simulink subsystem "Tranfsform_Linear_Gains_To_World"  (R2023a)
settings: Solver=VariableStepAuto  StartTime=0.0  StopTime=10.0  RelTol=1e-3

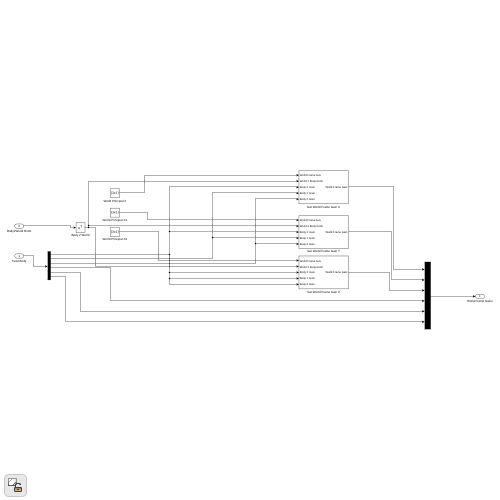
[thumbnail: Simulink's stored preview of the top-level diagram]
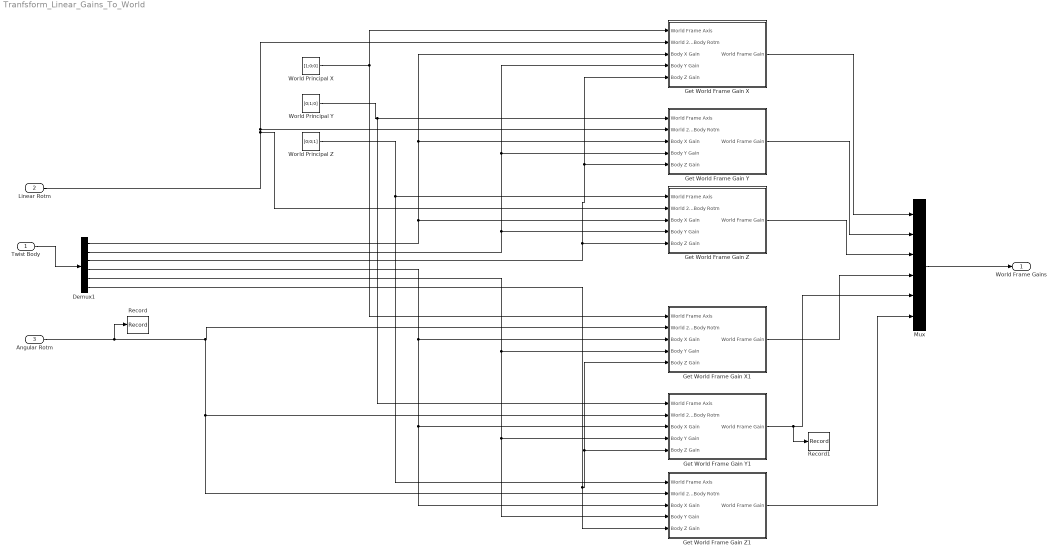
== system Tranfsform_Linear_Gains_To_World ==
  Twist Body : Inport
  Linear Rotm : Inport  Port=2
  Angular Rotm : Inport  Port=3
  Demux1 : Demux  Outputs=6
  Get World Frame Gain X : Subsystem
  Get World Frame Gain X1 : Subsystem
  Get World Frame Gain Y : Subsystem
  Get World Frame Gain Y1 : Subsystem
  Get World Frame Gain Z : Subsystem
  Get World Frame Gain Z1 : Subsystem
  Mux : Mux  Inputs=6
  Record : Record  FileSettingsInternal="{\"entries\":[{\"content\":{\"excelSettings\":{\"content\":{},\"type\":\"Streamout.ExcelSettings\"}},\"type\":\"Streamout.FileSettingStorage\",\"uuid\":\"\"}],\"packageUris\":[\"http:\\/\\/schema.mathworks.com\\/mf0\\/streamout_blocks\\/R2020a\"],\"version\":\"1.0\"}"  Layout=[1 1]  SignalsInternal="{\"entries\":[{\"content\":{\"signals\":[{\"content\":{\"blockPath\":[],\"dimensions\":[3,3],\"domain\":\"\",\"hasChildren\":true,\"lineColor\":\"#7e2f8e\",\"port\":1,\"signalID\":164792,\"signalName\":\"Angular Rotm\"},\"type\":\"RecordBlkView.Signal\",\"uuid\":\"\"},{\"content\":{\"blockPath\":[],\"channel\":[1,1],\"dimensions\":[3,3],\"domain\":\"\",\"lineColor\":\"#77ac30\",\"parentID\":164792,\"plots\":[1],\"port\":1,\"signalID\":164793,\"signalName\":\"An ...(+1923 chars)"  VisualizationBindings="{\"sparklinesplugin\":{\"info\":[{\"bindingParametersList\":[],\"subplotID\":1}]}}"
  Record1 : Record  FileSettingsInternal="{\"entries\":[{\"content\":{\"excelSettings\":{\"content\":{},\"type\":\"Streamout.ExcelSettings\"}},\"type\":\"Streamout.FileSettingStorage\",\"uuid\":\"\"}],\"packageUris\":[\"http:\\/\\/schema.mathworks.com\\/mf0\\/streamout_blocks\\/R2020a\"],\"version\":\"1.0\"}"  Layout=[1 1]  SignalsInternal="{\"entries\":[{\"content\":{\"signals\":[{\"content\":{\"blockPath\":[],\"dimensions\":[1],\"domain\":\"\",\"lineColor\":\"#a2142f\",\"plots\":[1],\"port\":1,\"signalID\":164815,\"signalName\":\"Get World Frame Gain Y1\"},\"type\":\"RecordBlkView.Signal\",\"uuid\":\"\"}]},\"type\":\"RecordBlkView.InputSignals\",\"uuid\":\"\"}],\"packageUris\":[\"http:\\/\\/schema.mathworks.com\\/mf0\\/streamout_blocks\\/R2020a\"],\"version\":\"1.0\"}"  VisualizationBindings="{\"sparklinesplugin\":{\"info\":[{\"bindingParametersList\":[],\"subplotID\":1}]}}"
  World Principal X : Constant  Value=[1;0;0]
  World Principal Y : Constant  Value=[0;1;0]
  World Principal Z : Constant  Value=[0;0;1]
  World Frame Gains : Outport
  wires:
  Twist Body/1 -> Demux1/1
  Demux1/1 -> Get World Frame Gain X/3(Body X Gain), Get World Frame Gain Y/3(Body X Gain), Get World Frame Gain Z/3(Body X Gain)
  Demux1/2 -> Get World Frame Gain X/4(Body Y Gain), Get World Frame Gain Y/4(Body Y Gain), Get World Frame Gain Z/4(Body Y Gain)
  Demux1/3 -> Get World Frame Gain X/5(Body Z Gain), Get World Frame Gain Y/5(Body Z Gain), Get World Frame Gain Z/5(Body Z Gain)
  Linear Rotm/1 -> Get World Frame Gain X/2(World 2 Body Rotm), Get World Frame Gain Y/2(World 2 Body Rotm), Get World Frame Gain Z/2(World 2 Body Rotm)
  Mux/1 -> World Frame Gains/1
  Get World Frame Gain X/1(World Frame Gain) -> Mux/1
  Get World Frame Gain Y/1(World Frame Gain) -> Mux/2
  Get World Frame Gain Z/1(World Frame Gain) -> Mux/3
  Get World Frame Gain Y1/1(World Frame Gain) -> Mux/5, Record1/1
  Demux1/5 -> Get World Frame Gain Y1/4(Body Y Gain), Get World Frame Gain Z1/4(Body Y Gain), Get World Frame Gain X1/4(Body Y Gain)
  Demux1/4 -> Get World Frame Gain Y1/3(Body X Gain), Get World Frame Gain Z1/3(Body X Gain), Get World Frame Gain X1/3(Body X Gain)
  World Principal Z/1 -> Get World Frame Gain Z/1(World Frame Axis), Get World Frame Gain Z1/1(World Frame Axis)
  World Principal X/1 -> Get World Frame Gain X1/1(World Frame Axis), Get World Frame Gain X/1(World Frame Axis)
  Get World Frame Gain Z1/1(World Frame Gain) -> Mux/6
  World Principal Y/1 -> Get World Frame Gain Y1/1(World Frame Axis), Get World Frame Gain Y/1(World Frame Axis)
  Demux1/6 -> Get World Frame Gain Y1/5(Body Z Gain), Get World Frame Gain X1/5(Body Z Gain), Get World Frame Gain Z1/5(Body Z Gain)
  Get World Frame Gain X1/1(World Frame Gain) -> Mux/4
  Angular Rotm/1 -> Get World Frame Gain Y1/2(World 2 Body Rotm), Get World Frame Gain Z1/2(World 2 Body Rotm), Get World Frame Gain X1/2(World 2 Body Rotm), Record/1

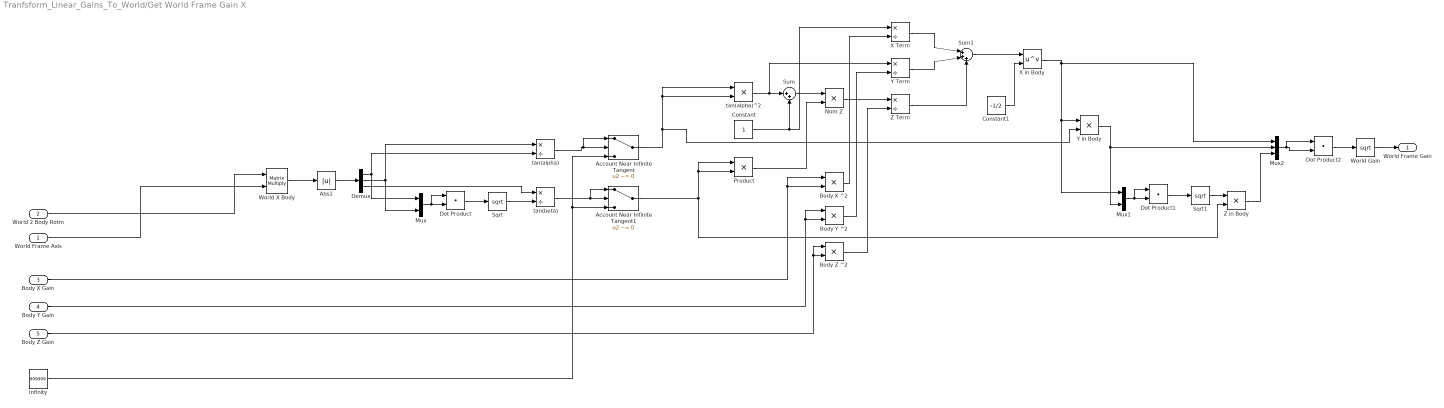
== system Tranfsform_Linear_Gains_To_World/Get World Frame Gain X ==
  World Frame Axis : Inport
  World 2 Body Rotm : Inport  Port=2
  Body X Gain : Inport  Port=3
  Body Y Gain : Inport  Port=4
  Body Z Gain : Inport  Port=5
  Abs1 : Abs  SaturateOnIntegerOverflow=off
  Account Near Infinite Tangent : Switch  Criteria=u2 ~= 0  SaturateOnIntegerOverflow=off  InputSameDT=off
  Account Near Infinite Tangent1 : Switch  Criteria=u2 ~= 0  SaturateOnIntegerOverflow=off  InputSameDT=off
  Body X ^2 : Product
  Body Y ^2 : Product
  Body Z ^2 : Product
  Constant : Constant
  Constant1 : Constant  Value=-1/2
  Demux : Demux  Outputs=3
  Dot Product : DotProduct  OutDataTypeStr=Inherit: Inherit via internal rule
  Dot Product1 : DotProduct  OutDataTypeStr=Inherit: Inherit via internal rule
  Dot Product2 : DotProduct  OutDataTypeStr=Inherit: Inherit via internal rule
  Infinity : Constant  Value=999999
  Mux : Mux  Inputs=2
  Mux1 : Mux  Inputs=2
  Mux2 : Mux  Inputs=3
  Num Z : Product
  Product : Product
  Sqrt : Sqrt
  Sqrt1 : Sqrt
  Sum : Sum  Inputs=|++
  Sum1 : Sum  Inputs=|+++
  World Gain : Sqrt
  World X Body : Product  Multiplication=Matrix(*)
  X Term : Product  Inputs=*/
  X in Body : Math  Operator=pow
  Y Term : Product  Inputs=*/
  Y in Body : Product
  Z Term : Product  Inputs=*/
  Z in Body : Product
  tan(alpha) : Product  Inputs=*/
  tan(alpha)^2 : Product
  tan(beta) : Product  Inputs=*/
  World Frame Gain : Outport
  wires:
  Account Near Infinite Tangent1/1 -> Z in Body/2, Product/1, Product/2
  tan(beta)/1 -> Account Near Infinite Tangent1/2, Account Near Infinite Tangent1/1
  Infinity/1 -> Account Near Infinite Tangent/3, Account Near Infinite Tangent1/3
  tan(alpha)/1 -> Account Near Infinite Tangent/2, Account Near Infinite Tangent/1
  Account Near Infinite Tangent/1 -> Y in Body/2, tan(alpha)^2/2, tan(alpha)^2/1
  World X Body/1 -> Abs1/1
  Sum/1 -> Num Z/1
  Mux2/1 -> Dot Product2/2, Dot Product2/1
  Demux/2 -> tan(alpha)/1, Mux/2
  Dot Product1/1 -> Sqrt1/1
  Constant/1 -> Sum/2, X Term/1
  Z in Body/1 -> Mux2/3
  Body X ^2/1 -> X Term/2
  Body X Gain/1 -> Body X ^2/1, Body X ^2/2
  Product/1 -> Num Z/2
  X Term/1 -> Sum1/1
  Abs1/1 -> Demux/1
  Dot Product/1 -> Sqrt/1
  Y Term/1 -> Sum1/2
  Body Z Gain/1 -> Body Z ^2/1, Body Z ^2/2
  Sqrt/1 -> tan(beta)/2
  Y in Body/1 -> Mux1/2, Mux2/2
  Sqrt1/1 -> Z in Body/1
  Body Y Gain/1 -> Body Y ^2/1, Body Y ^2/2
  Demux/1 -> tan(alpha)/2, Mux/1
  Body Z ^2/1 -> Z Term/2
  Num Z/1 -> Z Term/1
  Body Y ^2/1 -> Y Term/2
  X in Body/1 -> Y in Body/1, Mux1/1, Mux2/1
  Mux/1 -> Dot Product/1, Dot Product/2
  Constant1/1 -> X in Body/2
  Z Term/1 -> Sum1/3
  World Gain/1 -> World Frame Gain/1
  tan(alpha)^2/1 -> Sum/1, Y Term/1
  World 2 Body Rotm/1 -> World X Body/1
  Mux1/1 -> Dot Product1/1, Dot Product1/2
  Sum1/1 -> X in Body/1
  Dot Product2/1 -> World Gain/1
  World Frame Axis/1 -> World X Body/2
  Demux/3 -> tan(beta)/1

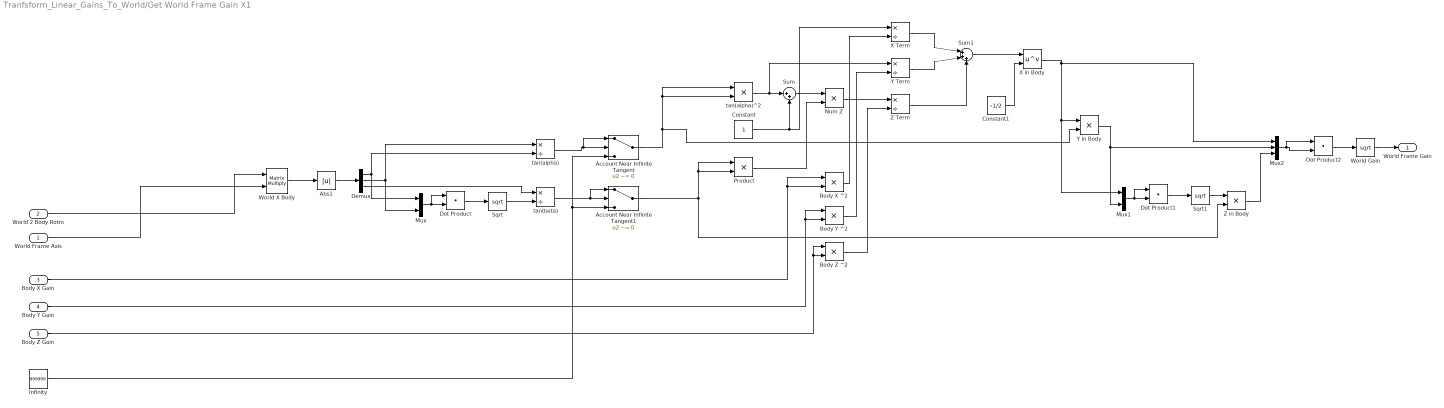
== system Tranfsform_Linear_Gains_To_World/Get World Frame Gain X1 ==
  World Frame Axis : Inport
  World 2 Body Rotm : Inport  Port=2
  Body X Gain : Inport  Port=3
  Body Y Gain : Inport  Port=4
  Body Z Gain : Inport  Port=5
  Abs1 : Abs  SaturateOnIntegerOverflow=off
  Account Near Infinite Tangent : Switch  Criteria=u2 ~= 0  SaturateOnIntegerOverflow=off  InputSameDT=off
  Account Near Infinite Tangent1 : Switch  Criteria=u2 ~= 0  SaturateOnIntegerOverflow=off  InputSameDT=off
  Body X ^2 : Product
  Body Y ^2 : Product
  Body Z ^2 : Product
  Constant : Constant
  Constant1 : Constant  Value=-1/2
  Demux : Demux  Outputs=3
  Dot Product : DotProduct  OutDataTypeStr=Inherit: Inherit via internal rule
  Dot Product1 : DotProduct  OutDataTypeStr=Inherit: Inherit via internal rule
  Dot Product2 : DotProduct  OutDataTypeStr=Inherit: Inherit via internal rule
  Infinity : Constant  Value=999999
  Mux : Mux  Inputs=2
  Mux1 : Mux  Inputs=2
  Mux2 : Mux  Inputs=3
  Num Z : Product
  Product : Product
  Sqrt : Sqrt
  Sqrt1 : Sqrt
  Sum : Sum  Inputs=|++
  Sum1 : Sum  Inputs=|+++
  World Gain : Sqrt
  World X Body : Product  Multiplication=Matrix(*)
  X Term : Product  Inputs=*/
  X in Body : Math  Operator=pow
  Y Term : Product  Inputs=*/
  Y in Body : Product
  Z Term : Product  Inputs=*/
  Z in Body : Product
  tan(alpha) : Product  Inputs=*/
  tan(alpha)^2 : Product
  tan(beta) : Product  Inputs=*/
  World Frame Gain : Outport
  wires:
  Account Near Infinite Tangent1/1 -> Z in Body/2, Product/1, Product/2
  tan(beta)/1 -> Account Near Infinite Tangent1/2, Account Near Infinite Tangent1/1
  Infinity/1 -> Account Near Infinite Tangent/3, Account Near Infinite Tangent1/3
  tan(alpha)/1 -> Account Near Infinite Tangent/2, Account Near Infinite Tangent/1
  Account Near Infinite Tangent/1 -> Y in Body/2, tan(alpha)^2/2, tan(alpha)^2/1
  World X Body/1 -> Abs1/1
  Sum/1 -> Num Z/1
  Mux2/1 -> Dot Product2/2, Dot Product2/1
  Demux/2 -> tan(alpha)/1, Mux/2
  Dot Product1/1 -> Sqrt1/1
  Constant/1 -> Sum/2, X Term/1
  Z in Body/1 -> Mux2/3
  Body X ^2/1 -> X Term/2
  Body X Gain/1 -> Body X ^2/1, Body X ^2/2
  Product/1 -> Num Z/2
  X Term/1 -> Sum1/1
  Abs1/1 -> Demux/1
  Dot Product/1 -> Sqrt/1
  Y Term/1 -> Sum1/2
  Body Z Gain/1 -> Body Z ^2/1, Body Z ^2/2
  Sqrt/1 -> tan(beta)/2
  Y in Body/1 -> Mux1/2, Mux2/2
  Sqrt1/1 -> Z in Body/1
  Body Y Gain/1 -> Body Y ^2/1, Body Y ^2/2
  Demux/1 -> tan(alpha)/2, Mux/1
  Body Z ^2/1 -> Z Term/2
  Num Z/1 -> Z Term/1
  Body Y ^2/1 -> Y Term/2
  X in Body/1 -> Y in Body/1, Mux1/1, Mux2/1
  Mux/1 -> Dot Product/1, Dot Product/2
  Constant1/1 -> X in Body/2
  Z Term/1 -> Sum1/3
  World Gain/1 -> World Frame Gain/1
  tan(alpha)^2/1 -> Sum/1, Y Term/1
  World 2 Body Rotm/1 -> World X Body/1
  Mux1/1 -> Dot Product1/1, Dot Product1/2
  Sum1/1 -> X in Body/1
  Dot Product2/1 -> World Gain/1
  World Frame Axis/1 -> World X Body/2
  Demux/3 -> tan(beta)/1

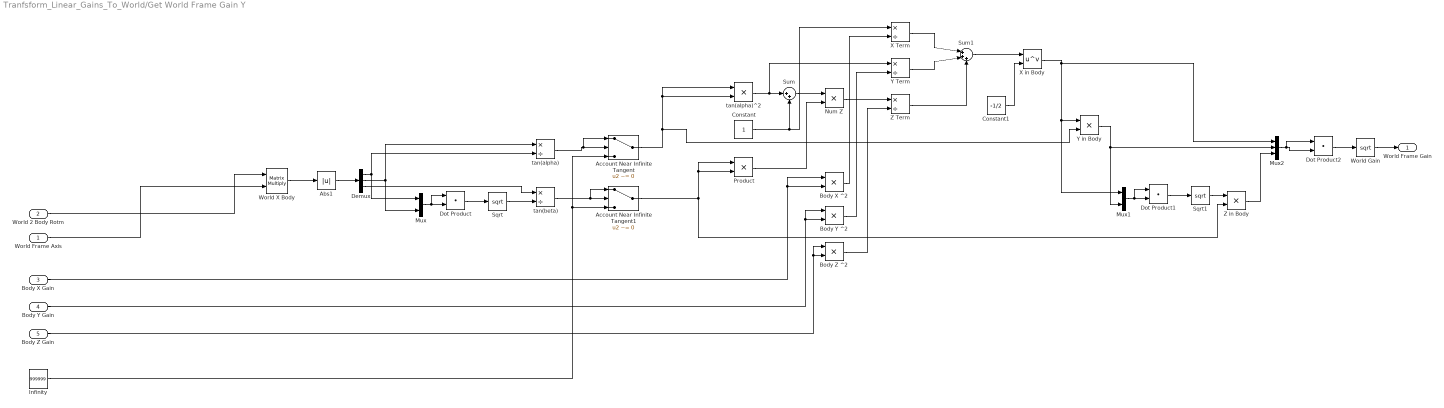
== system Tranfsform_Linear_Gains_To_World/Get World Frame Gain Y ==
  World Frame Axis : Inport
  World 2 Body Rotm : Inport  Port=2
  Body X Gain : Inport  Port=3
  Body Y Gain : Inport  Port=4
  Body Z Gain : Inport  Port=5
  Abs1 : Abs  SaturateOnIntegerOverflow=off
  Account Near Infinite Tangent : Switch  Criteria=u2 ~= 0  SaturateOnIntegerOverflow=off  InputSameDT=off
  Account Near Infinite Tangent1 : Switch  Criteria=u2 ~= 0  SaturateOnIntegerOverflow=off  InputSameDT=off
  Body X ^2 : Product
  Body Y ^2 : Product
  Body Z ^2 : Product
  Constant : Constant
  Constant1 : Constant  Value=-1/2
  Demux : Demux  Outputs=3
  Dot Product : DotProduct  OutDataTypeStr=Inherit: Inherit via internal rule
  Dot Product1 : DotProduct  OutDataTypeStr=Inherit: Inherit via internal rule
  Dot Product2 : DotProduct  OutDataTypeStr=Inherit: Inherit via internal rule
  Infinity : Constant  Value=999999
  Mux : Mux  Inputs=2
  Mux1 : Mux  Inputs=2
  Mux2 : Mux  Inputs=3
  Num Z : Product
  Product : Product
  Sqrt : Sqrt
  Sqrt1 : Sqrt
  Sum : Sum  Inputs=|++
  Sum1 : Sum  Inputs=|+++
  World Gain : Sqrt
  World X Body : Product  Multiplication=Matrix(*)
  X Term : Product  Inputs=*/
  X in Body : Math  Operator=pow
  Y Term : Product  Inputs=*/
  Y in Body : Product
  Z Term : Product  Inputs=*/
  Z in Body : Product
  tan(alpha) : Product  Inputs=*/
  tan(alpha)^2 : Product
  tan(beta) : Product  Inputs=*/
  World Frame Gain : Outport
  wires:
  Account Near Infinite Tangent1/1 -> Z in Body/2, Product/1, Product/2
  tan(beta)/1 -> Account Near Infinite Tangent1/2, Account Near Infinite Tangent1/1
  Infinity/1 -> Account Near Infinite Tangent/3, Account Near Infinite Tangent1/3
  tan(alpha)/1 -> Account Near Infinite Tangent/2, Account Near Infinite Tangent/1
  Account Near Infinite Tangent/1 -> Y in Body/2, tan(alpha)^2/2, tan(alpha)^2/1
  World X Body/1 -> Abs1/1
  Sum/1 -> Num Z/1
  Mux2/1 -> Dot Product2/2, Dot Product2/1
  Demux/2 -> tan(alpha)/1, Mux/2
  Dot Product1/1 -> Sqrt1/1
  Constant/1 -> Sum/2, X Term/1
  Z in Body/1 -> Mux2/3
  Body X ^2/1 -> X Term/2
  Body X Gain/1 -> Body X ^2/1, Body X ^2/2
  Product/1 -> Num Z/2
  X Term/1 -> Sum1/1
  Abs1/1 -> Demux/1
  Dot Product/1 -> Sqrt/1
  Y Term/1 -> Sum1/2
  Body Z Gain/1 -> Body Z ^2/1, Body Z ^2/2
  Sqrt/1 -> tan(beta)/2
  Y in Body/1 -> Mux1/2, Mux2/2
  Sqrt1/1 -> Z in Body/1
  Body Y Gain/1 -> Body Y ^2/1, Body Y ^2/2
  Demux/1 -> tan(alpha)/2, Mux/1
  Body Z ^2/1 -> Z Term/2
  Num Z/1 -> Z Term/1
  Body Y ^2/1 -> Y Term/2
  X in Body/1 -> Y in Body/1, Mux1/1, Mux2/1
  Mux/1 -> Dot Product/1, Dot Product/2
  Constant1/1 -> X in Body/2
  Z Term/1 -> Sum1/3
  World Gain/1 -> World Frame Gain/1
  tan(alpha)^2/1 -> Sum/1, Y Term/1
  World 2 Body Rotm/1 -> World X Body/1
  Mux1/1 -> Dot Product1/1, Dot Product1/2
  Sum1/1 -> X in Body/1
  Dot Product2/1 -> World Gain/1
  World Frame Axis/1 -> World X Body/2
  Demux/3 -> tan(beta)/1

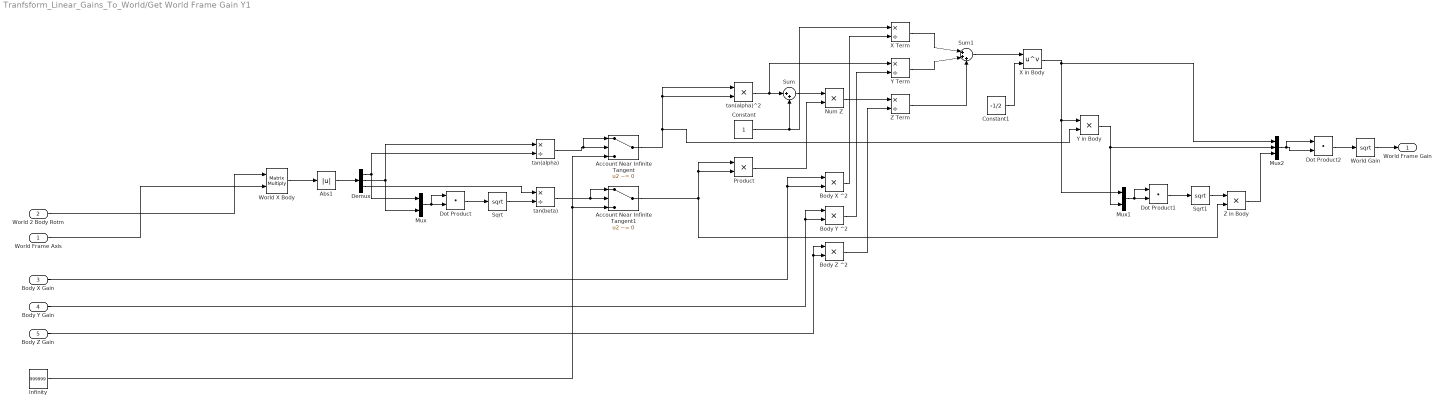
== system Tranfsform_Linear_Gains_To_World/Get World Frame Gain Y1 ==
  World Frame Axis : Inport
  World 2 Body Rotm : Inport  Port=2
  Body X Gain : Inport  Port=3
  Body Y Gain : Inport  Port=4
  Body Z Gain : Inport  Port=5
  Abs1 : Abs  SaturateOnIntegerOverflow=off
  Account Near Infinite Tangent : Switch  Criteria=u2 ~= 0  SaturateOnIntegerOverflow=off  InputSameDT=off
  Account Near Infinite Tangent1 : Switch  Criteria=u2 ~= 0  SaturateOnIntegerOverflow=off  InputSameDT=off
  Body X ^2 : Product
  Body Y ^2 : Product
  Body Z ^2 : Product
  Constant : Constant
  Constant1 : Constant  Value=-1/2
  Demux : Demux  Outputs=3
  Dot Product : DotProduct  OutDataTypeStr=Inherit: Inherit via internal rule
  Dot Product1 : DotProduct  OutDataTypeStr=Inherit: Inherit via internal rule
  Dot Product2 : DotProduct  OutDataTypeStr=Inherit: Inherit via internal rule
  Infinity : Constant  Value=999999
  Mux : Mux  Inputs=2
  Mux1 : Mux  Inputs=2
  Mux2 : Mux  Inputs=3
  Num Z : Product
  Product : Product
  Sqrt : Sqrt
  Sqrt1 : Sqrt
  Sum : Sum  Inputs=|++
  Sum1 : Sum  Inputs=|+++
  World Gain : Sqrt
  World X Body : Product  Multiplication=Matrix(*)
  X Term : Product  Inputs=*/
  X in Body : Math  Operator=pow
  Y Term : Product  Inputs=*/
  Y in Body : Product
  Z Term : Product  Inputs=*/
  Z in Body : Product
  tan(alpha) : Product  Inputs=*/
  tan(alpha)^2 : Product
  tan(beta) : Product  Inputs=*/
  World Frame Gain : Outport
  wires:
  Account Near Infinite Tangent1/1 -> Z in Body/2, Product/1, Product/2
  tan(beta)/1 -> Account Near Infinite Tangent1/2, Account Near Infinite Tangent1/1
  Infinity/1 -> Account Near Infinite Tangent/3, Account Near Infinite Tangent1/3
  tan(alpha)/1 -> Account Near Infinite Tangent/2, Account Near Infinite Tangent/1
  Account Near Infinite Tangent/1 -> Y in Body/2, tan(alpha)^2/2, tan(alpha)^2/1
  World X Body/1 -> Abs1/1
  Sum/1 -> Num Z/1
  Mux2/1 -> Dot Product2/2, Dot Product2/1
  Demux/2 -> tan(alpha)/1, Mux/2
  Dot Product1/1 -> Sqrt1/1
  Constant/1 -> Sum/2, X Term/1
  Z in Body/1 -> Mux2/3
  Body X ^2/1 -> X Term/2
  Body X Gain/1 -> Body X ^2/1, Body X ^2/2
  Product/1 -> Num Z/2
  X Term/1 -> Sum1/1
  Abs1/1 -> Demux/1
  Dot Product/1 -> Sqrt/1
  Y Term/1 -> Sum1/2
  Body Z Gain/1 -> Body Z ^2/1, Body Z ^2/2
  Sqrt/1 -> tan(beta)/2
  Y in Body/1 -> Mux1/2, Mux2/2
  Sqrt1/1 -> Z in Body/1
  Body Y Gain/1 -> Body Y ^2/1, Body Y ^2/2
  Demux/1 -> tan(alpha)/2, Mux/1
  Body Z ^2/1 -> Z Term/2
  Num Z/1 -> Z Term/1
  Body Y ^2/1 -> Y Term/2
  X in Body/1 -> Y in Body/1, Mux1/1, Mux2/1
  Mux/1 -> Dot Product/1, Dot Product/2
  Constant1/1 -> X in Body/2
  Z Term/1 -> Sum1/3
  World Gain/1 -> World Frame Gain/1
  tan(alpha)^2/1 -> Sum/1, Y Term/1
  World 2 Body Rotm/1 -> World X Body/1
  Mux1/1 -> Dot Product1/1, Dot Product1/2
  Sum1/1 -> X in Body/1
  Dot Product2/1 -> World Gain/1
  World Frame Axis/1 -> World X Body/2
  Demux/3 -> tan(beta)/1

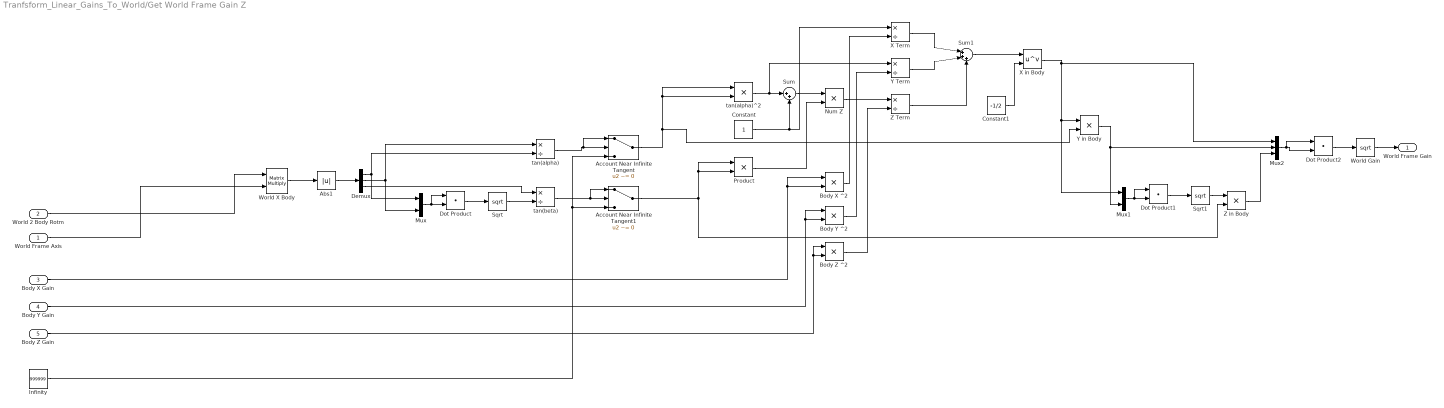
== system Tranfsform_Linear_Gains_To_World/Get World Frame Gain Z ==
  World Frame Axis : Inport
  World 2 Body Rotm : Inport  Port=2
  Body X Gain : Inport  Port=3
  Body Y Gain : Inport  Port=4
  Body Z Gain : Inport  Port=5
  Abs1 : Abs  SaturateOnIntegerOverflow=off
  Account Near Infinite Tangent : Switch  Criteria=u2 ~= 0  SaturateOnIntegerOverflow=off  InputSameDT=off
  Account Near Infinite Tangent1 : Switch  Criteria=u2 ~= 0  SaturateOnIntegerOverflow=off  InputSameDT=off
  Body X ^2 : Product
  Body Y ^2 : Product
  Body Z ^2 : Product
  Constant : Constant
  Constant1 : Constant  Value=-1/2
  Demux : Demux  Outputs=3
  Dot Product : DotProduct  OutDataTypeStr=Inherit: Inherit via internal rule
  Dot Product1 : DotProduct  OutDataTypeStr=Inherit: Inherit via internal rule
  Dot Product2 : DotProduct  OutDataTypeStr=Inherit: Inherit via internal rule
  Infinity : Constant  Value=999999
  Mux : Mux  Inputs=2
  Mux1 : Mux  Inputs=2
  Mux2 : Mux  Inputs=3
  Num Z : Product
  Product : Product
  Sqrt : Sqrt
  Sqrt1 : Sqrt
  Sum : Sum  Inputs=|++
  Sum1 : Sum  Inputs=|+++
  World Gain : Sqrt
  World X Body : Product  Multiplication=Matrix(*)
  X Term : Product  Inputs=*/
  X in Body : Math  Operator=pow
  Y Term : Product  Inputs=*/
  Y in Body : Product
  Z Term : Product  Inputs=*/
  Z in Body : Product
  tan(alpha) : Product  Inputs=*/
  tan(alpha)^2 : Product
  tan(beta) : Product  Inputs=*/
  World Frame Gain : Outport
  wires:
  Account Near Infinite Tangent1/1 -> Z in Body/2, Product/1, Product/2
  tan(beta)/1 -> Account Near Infinite Tangent1/2, Account Near Infinite Tangent1/1
  Infinity/1 -> Account Near Infinite Tangent/3, Account Near Infinite Tangent1/3
  tan(alpha)/1 -> Account Near Infinite Tangent/2, Account Near Infinite Tangent/1
  Account Near Infinite Tangent/1 -> Y in Body/2, tan(alpha)^2/2, tan(alpha)^2/1
  World X Body/1 -> Abs1/1
  Sum/1 -> Num Z/1
  Mux2/1 -> Dot Product2/2, Dot Product2/1
  Demux/2 -> tan(alpha)/1, Mux/2
  Dot Product1/1 -> Sqrt1/1
  Constant/1 -> Sum/2, X Term/1
  Z in Body/1 -> Mux2/3
  Body X ^2/1 -> X Term/2
  Body X Gain/1 -> Body X ^2/1, Body X ^2/2
  Product/1 -> Num Z/2
  X Term/1 -> Sum1/1
  Abs1/1 -> Demux/1
  Dot Product/1 -> Sqrt/1
  Y Term/1 -> Sum1/2
  Body Z Gain/1 -> Body Z ^2/1, Body Z ^2/2
  Sqrt/1 -> tan(beta)/2
  Y in Body/1 -> Mux1/2, Mux2/2
  Sqrt1/1 -> Z in Body/1
  Body Y Gain/1 -> Body Y ^2/1, Body Y ^2/2
  Demux/1 -> tan(alpha)/2, Mux/1
  Body Z ^2/1 -> Z Term/2
  Num Z/1 -> Z Term/1
  Body Y ^2/1 -> Y Term/2
  X in Body/1 -> Y in Body/1, Mux1/1, Mux2/1
  Mux/1 -> Dot Product/1, Dot Product/2
  Constant1/1 -> X in Body/2
  Z Term/1 -> Sum1/3
  World Gain/1 -> World Frame Gain/1
  tan(alpha)^2/1 -> Sum/1, Y Term/1
  World 2 Body Rotm/1 -> World X Body/1
  Mux1/1 -> Dot Product1/1, Dot Product1/2
  Sum1/1 -> X in Body/1
  Dot Product2/1 -> World Gain/1
  World Frame Axis/1 -> World X Body/2
  Demux/3 -> tan(beta)/1

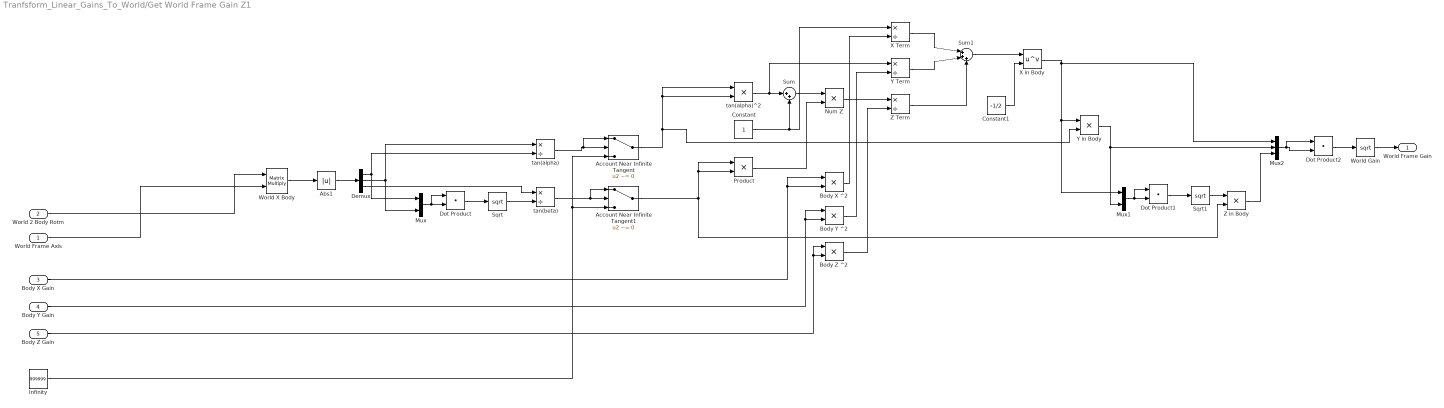
== system Tranfsform_Linear_Gains_To_World/Get World Frame Gain Z1 ==
  World Frame Axis : Inport
  World 2 Body Rotm : Inport  Port=2
  Body X Gain : Inport  Port=3
  Body Y Gain : Inport  Port=4
  Body Z Gain : Inport  Port=5
  Abs1 : Abs  SaturateOnIntegerOverflow=off
  Account Near Infinite Tangent : Switch  Criteria=u2 ~= 0  SaturateOnIntegerOverflow=off  InputSameDT=off
  Account Near Infinite Tangent1 : Switch  Criteria=u2 ~= 0  SaturateOnIntegerOverflow=off  InputSameDT=off
  Body X ^2 : Product
  Body Y ^2 : Product
  Body Z ^2 : Product
  Constant : Constant
  Constant1 : Constant  Value=-1/2
  Demux : Demux  Outputs=3
  Dot Product : DotProduct  OutDataTypeStr=Inherit: Inherit via internal rule
  Dot Product1 : DotProduct  OutDataTypeStr=Inherit: Inherit via internal rule
  Dot Product2 : DotProduct  OutDataTypeStr=Inherit: Inherit via internal rule
  Infinity : Constant  Value=999999
  Mux : Mux  Inputs=2
  Mux1 : Mux  Inputs=2
  Mux2 : Mux  Inputs=3
  Num Z : Product
  Product : Product
  Sqrt : Sqrt
  Sqrt1 : Sqrt
  Sum : Sum  Inputs=|++
  Sum1 : Sum  Inputs=|+++
  World Gain : Sqrt
  World X Body : Product  Multiplication=Matrix(*)
  X Term : Product  Inputs=*/
  X in Body : Math  Operator=pow
  Y Term : Product  Inputs=*/
  Y in Body : Product
  Z Term : Product  Inputs=*/
  Z in Body : Product
  tan(alpha) : Product  Inputs=*/
  tan(alpha)^2 : Product
  tan(beta) : Product  Inputs=*/
  World Frame Gain : Outport
  wires:
  Account Near Infinite Tangent1/1 -> Z in Body/2, Product/1, Product/2
  tan(beta)/1 -> Account Near Infinite Tangent1/2, Account Near Infinite Tangent1/1
  Infinity/1 -> Account Near Infinite Tangent/3, Account Near Infinite Tangent1/3
  tan(alpha)/1 -> Account Near Infinite Tangent/2, Account Near Infinite Tangent/1
  Account Near Infinite Tangent/1 -> Y in Body/2, tan(alpha)^2/2, tan(alpha)^2/1
  World X Body/1 -> Abs1/1
  Sum/1 -> Num Z/1
  Mux2/1 -> Dot Product2/2, Dot Product2/1
  Demux/2 -> tan(alpha)/1, Mux/2
  Dot Product1/1 -> Sqrt1/1
  Constant/1 -> Sum/2, X Term/1
  Z in Body/1 -> Mux2/3
  Body X ^2/1 -> X Term/2
  Body X Gain/1 -> Body X ^2/1, Body X ^2/2
  Product/1 -> Num Z/2
  X Term/1 -> Sum1/1
  Abs1/1 -> Demux/1
  Dot Product/1 -> Sqrt/1
  Y Term/1 -> Sum1/2
  Body Z Gain/1 -> Body Z ^2/1, Body Z ^2/2
  Sqrt/1 -> tan(beta)/2
  Y in Body/1 -> Mux1/2, Mux2/2
  Sqrt1/1 -> Z in Body/1
  Body Y Gain/1 -> Body Y ^2/1, Body Y ^2/2
  Demux/1 -> tan(alpha)/2, Mux/1
  Body Z ^2/1 -> Z Term/2
  Num Z/1 -> Z Term/1
  Body Y ^2/1 -> Y Term/2
  X in Body/1 -> Y in Body/1, Mux1/1, Mux2/1
  Mux/1 -> Dot Product/1, Dot Product/2
  Constant1/1 -> X in Body/2
  Z Term/1 -> Sum1/3
  World Gain/1 -> World Frame Gain/1
  tan(alpha)^2/1 -> Sum/1, Y Term/1
  World 2 Body Rotm/1 -> World X Body/1
  Mux1/1 -> Dot Product1/1, Dot Product1/2
  Sum1/1 -> X in Body/1
  Dot Product2/1 -> World Gain/1
  World Frame Axis/1 -> World X Body/2
  Demux/3 -> tan(beta)/1
